simulink model "model7Krata"  (Simulink 6.6)
settings: Solver=ode45  StartTime=0.0  StopTime=700  MaxStep=0.01  MinStep=0.001  RelTol=1e-6
values from neighbouring files (symbols this model uses):
  c1 = 8    [dane7Krata.m]
  c2 = 5    [dane7Krata.m]
  E = 0.1*h2    (= 0.4)    [dane7Krata.m]
  h1 = (mi1*mi1+mi2*mi2)*q*q    (= 5)    [dane7Krata.m]
  h2 = mi2*mi2*q*q    (= 4)    [dane7Krata.m]
  mi1 = 1    [dane7Krata.m]
  mi2 = 2    [dane7Krata.m]
  p0 = h2    (= 4)    [dane7Krata.m]
undefined symbols (not defined in the file or in its folder): sgn
settings Model: Creator=Administrator  LastModifiedBy=Damian
settings DataIOCC: LimitDataPoints=off
settings GRTTargetCC: TargetFcnLib=ansi_tfl_table_tmw.mat

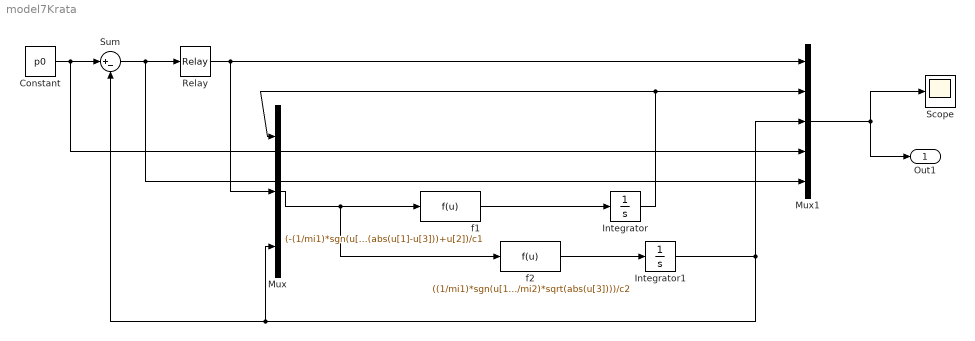
== system model7Krata ==
  Constant : Constant  Value=p0
  Integrator : Integrator  InitialCondition=h1
  Integrator1 : Integrator  InitialCondition=h2
  Mux : Mux  Inputs=3
  Mux1 : Mux  Inputs=5
  Relay : Relay  OnSwitchValue=E  OffSwitchValue=-E  OnOutputValue=U
  Scope : Scope
      settings: YMin=0
  Sum : Sum  Inputs=|+-
  f1 : Fcn  Tag=f1  Expr=(-(1/mi1)*sgn(u[1]-u[3])*sqrt(abs(u[1]-u[3]))+u[2])/c1
  f2 : Fcn  Expr=((1/mi1)*sgn(u[1]-u[3])*sqrt(abs(u[1]-u[3]))-(1/mi2)*sqrt(abs(u[3])))/c2
  Out1 : Outport
  wires:
  Mux/1 -> f1/1, f2/1
  f2/1 -> Integrator1/1
  f1/1 -> Integrator/1
  Integrator/1 -> Mux/1, Mux1/2
  Integrator1/1 -> Mux1/3, Mux/3, Sum/2
  Mux1/1 -> Scope/1, Out1/1
  Constant/1 -> Sum/1, Mux1/4
  Sum/1 -> Relay/1, Mux1/5
  Relay/1 -> Mux1/1, Mux/2
